simulink model "ModMarzo2023"  (R2019a)
settings: Solver=VariableStepAuto  StartTime=0.0  StopTime=1000  MaxStep=0.001  RelTol=1e-3
values from neighbouring files (symbols this model uses):
  K1 = 0.7    [InterpPesosPartesEDOs.m]
  K2 = 0.036893    [InterpPesosPartesEDOs.m]
  K3 = ((44.75-19)/515)    (= 0.05)    [InterpPesosPartesEDOs.m]
libraries: simulink x1
settings Model: Creator=Luis F Guevara G  LastModifiedBy=Luis F Guevara G

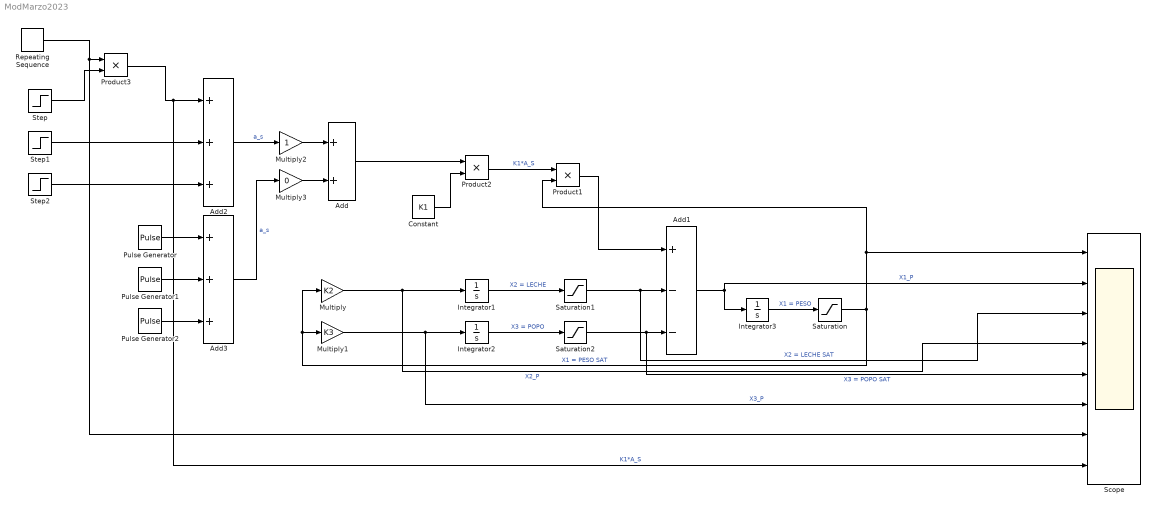
== system ModMarzo2023 ==
  Add : Sum
  Add1 : Sum  Inputs=+--
  Add2 : Sum  Inputs=+++
  Add3 : Sum  Inputs=+++
  Constant : Constant  Value=K1
  Integrator1 : Integrator  InitialCondition=19
  Integrator2 : Integrator  InitialCondition=25.75
  Integrator3 : Integrator  InitialCondition=515
  Multiply : Gain  Gain=K2
  Multiply1 : Gain  Gain=K3
  Multiply2 : Gain
  Multiply3 : Gain  Gain=0
  Product1 : Product
  Product2 : Product
  Product3 : Product
  Pulse Generator : DiscretePulseGenerator  PulseType=Time based  Amplitude=0.2  Period=50  PulseWidth=25
  Pulse Generator1 : DiscretePulseGenerator  PulseType=Time based  Amplitude=0.04  Period=50  PulseWidth=25
  Pulse Generator2 : DiscretePulseGenerator  PulseType=Time based  Amplitude=0.1  Period=50  PulseWidth=25
  Repeating Sequence : simulink/Sources/Repeating Sequence  rep_seq_t=P3FER_T  rep_seq_y=P3FER_W
  Saturation : Saturate  UpperLimit=630  LowerLimit=470
  Saturation1 : Saturate  UpperLimit=40  LowerLimit=5
  Saturation2 : Saturate  UpperLimit=35  LowerLimit=5
  Scope : Scope  NumInputPorts=8
  Step : Step  Time=0  Before=0.2  After=0.2  SampleTime=0
  Step1 : Step  Time=0  Before=0.04  After=0  SampleTime=0
  Step2 : Step  Time=0  Before=0.1  After=0  SampleTime=0
  wires:
  Step/1 -> Product3/2
  Step1/1 -> Add2/2
  Step2/1 -> Add2/3
  Integrator3/1 -> Saturation/1  "X1 = PESO"
  Product1/1 -> Add1/1
  Add1/1 -> Integrator3/1, Scope/2  "X1_P"
  Multiply/1 -> Integrator1/1, Scope/4  "X2_P"
  Multiply1/1 -> Integrator2/1, Scope/6  "X3_P"
  Integrator1/1 -> Saturation1/1  "X2 = LECHE"
  Integrator2/1 -> Saturation2/1  "X3 = POPO"
  Add2/1 -> Multiply2/1  "a_s"
  Product2/1 -> Product1/1  "K1*A_S"
  Constant/1 -> Product2/2
  Saturation/1 -> Multiply/1, Multiply1/1, Product1/2, Scope/1  "X1 = PESO SAT"
  Saturation1/1 -> Scope/3, Add1/2  "X2 = LECHE SAT"
  Saturation2/1 -> Scope/5, Add1/3  "X3 = POPO SAT"
  Pulse Generator2/1 -> Add3/3
  Pulse Generator1/1 -> Add3/2
  Pulse Generator/1 -> Add3/1
  Multiply3/1 -> Add/2
  Multiply2/1 -> Add/1
  Add/1 -> Product2/1
  Add3/1 -> Multiply3/1  "a_s"
  Repeating Sequence/1 -> Product3/1, Scope/7
  Product3/1 -> Scope/8, Add2/1  "K1*A_S"
